simulink model "Experiment_Qcar_Nonlinear_MPC"  (R2024b)
settings: Solver=ode2  StartTime=0.0  StopTime=Tf  FixedStep=Ts2  RelTol=1e-3  EnableMultiTasking=on
values from neighbouring files (symbols this model uses):
  alpha_kalman = 0.9    [setup_FL_MPC.m]    (also in setup_NL_MPC.m; setup_backstepping.m)
  beta_kalman = 2    [setup_FL_MPC.m]    (also in setup_NL_MPC.m; setup_backstepping.m)
  kappa_kalman = 0    [setup_FL_MPC.m]    (also in setup_NL_MPC.m; setup_backstepping.m)
  l = 0.256    [setup_FL_MPC.m]    (also in setup_NL_MPC.m; setup_backstepping.m)
  N = 10    [setup_FL_MPC.m]    (also in setup_NL_MPC.m; setup_backstepping.m = 5)
  P0_kalman = diag([1e-5 1e-5 1e-6 1e-6])    [setup_FL_MPC.m]    (also in setup_NL_MPC.m; setup_backstepping.m)
  q0 = [x0;y0;theta0;0]    [setup_FL_MPC.m]    (also in setup_NL_MPC.m; setup_backstepping.m)
  Q_kalman = diag([0.001 0.001 0.1 1])    [setup_FL_MPC.m]    (also in setup_NL_MPC.m = diag([0.001 0.001 0.1 10]); setup_backstepping.m = diag([0.001 0.001 0.1 10]))
  Qhat = qz*eye(2*N)    [setup_FL_MPC.m]    (also in setup_NL_MPC.m = blkdiag(Qhat,Q))
  R_kalman = diag([2e-5 2e-5 0.0001 0.001])    [setup_FL_MPC.m]    (also in setup_NL_MPC.m = diag([2e-5 2e-5 0.0001 0.00001]); setup_backstepping.m = diag([2e-5 2e-5 0.0001 0.00001]))
  Rhat = qu*eye(2*N)    [setup_FL_MPC.m]    (also in setup_NL_MPC.m = blkdiag(Rhat,R))
  theta0 = vicon_data(6)    [setup_FL_MPC.m]    (also in setup_NL_MPC.m; setup_backstepping.m)
  Ts = 0.008    [setup_FL_MPC.m]    (also in setup_NL_MPC.m = 0.01; setup_backstepping.m = 0.1)
  Ts2 = Ts    (= 0.008)    [setup_FL_MPC.m]    (also in setup_NL_MPC.m = 0.01; setup_backstepping.m = 0.1)
  v1max = 1    [setup_FL_MPC.m]    (also in setup_NL_MPC.m; setup_backstepping.m)
  v2max = 10    [setup_FL_MPC.m]    (also in setup_NL_MPC.m; setup_backstepping.m)
  x0 = vicon_data(1)    [setup_FL_MPC.m]    (also in setup_NL_MPC.m; setup_backstepping.m)
  y0 = vicon_data(2)    [setup_FL_MPC.m]    (also in setup_NL_MPC.m; setup_backstepping.m)
undefined symbols (not defined in the file or in its folder): DiscIntNeverNeededParam, HIL
libraries: quarc_library x16, simulink x2, dspsigops x1, slpidlib x1
settings Model: SimulationMode=external  ExtModeTrigDuration=10000  Creator=mbohra  LastModifiedBy=tirio
settings SolverCC: AlgebraicLoopSolver=TrustRegion  PositivePriorityOrder=on  AutoInsertRateTranBlk=on
settings DataIOCC: SaveOutput=off  SignalLogging=off  DSMLogging=off  SaveTime=off  ReturnWorkspaceOutputs=off
settings OptimizationCC: ReuseModelBlockBuffer=off
settings DebuggingCC: UnconnectedInputMsg=warning  UnconnectedOutputMsg=warning  UnconnectedLineMsg=warning  ArithmeticOperatorsInVariantConditions=warning
settings HardwareCC: ProdBitPerLong=64  ProdLargestAtomicInteger=LongLong  ProdLargestAtomicFloat=Double  ProdLongLongMode=on  ProdHWDeviceType=ARM Compatible->ARM 64-bit (LP64)
settings ModelReferenceCC: EnableRefExpFcnMdlSchedulingChecks=on
settings SFSimCC: CustomCodeUndefinedFunction=UseInterfaceOnly
settings RTWCC: Description=QUARC Linux Nvidia Target (QCar) Using Toolchain  SystemTargetFile=quarc_linux_nvidia.tlc  TemplateMakefile=quarc_default_tmf  Toolchain=QUARC linux_nvidia | gmake (64-bit Windows)  BuildConfiguration=Faster Runs  GPUComputeCapability=3.5  DLArmComputeVersion=19.05
settings STFCustomTargetCC: TargetLangStandard=C99 (ISO)  ConcurrentExecutionCompliant=on  GRTInterface=on  UseToolchainInfoCompliant=on  SystemTargetFile=quarc_linux_nvidia.tlc
settings GRTTargetCC: ParMdlRefBuildCompliant=off  CompOptLevelCompliant=off  CombineOutputUpdateFcns=off  MatFileLogging=off  CPPClassGenCompliant=off  GRTInterface=on  ExtMode=on  ExtModeMexFile=quarc_comm  ExtModeMexArgs='-w -d /tmp -uri %u','tcpip://192.168.0.143:17001'

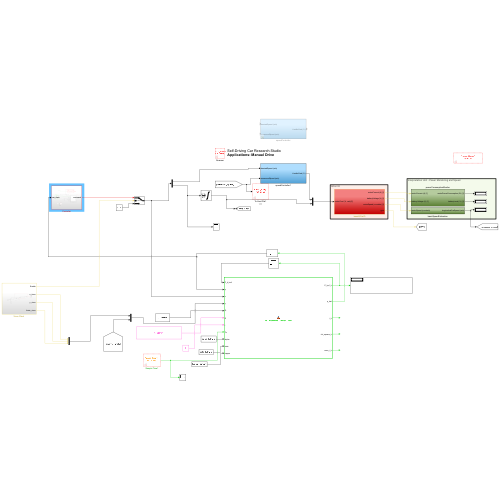
[thumbnail: Simulink's stored preview of the top-level diagram]
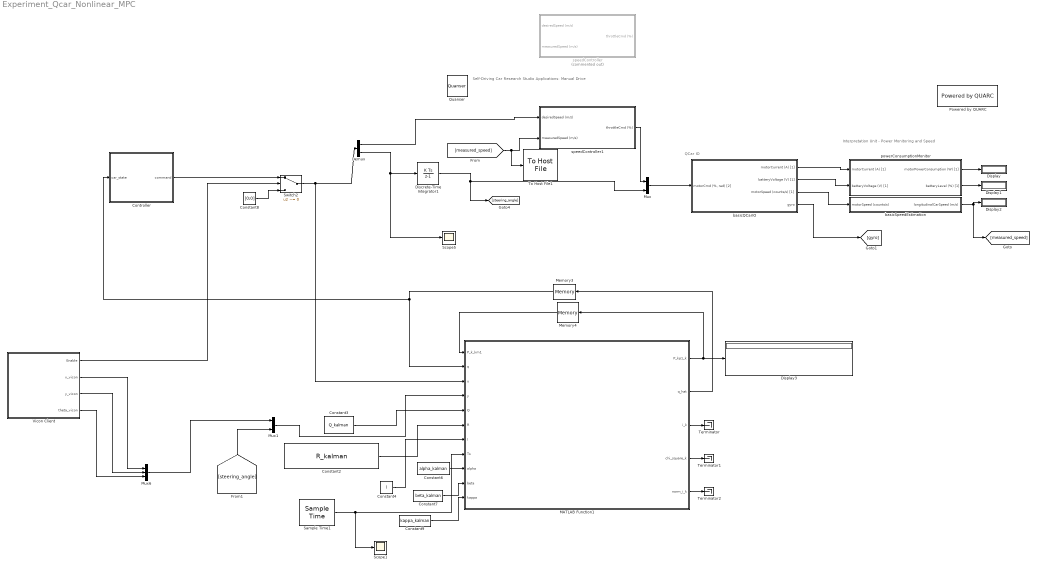
== system Experiment_Qcar_Nonlinear_MPC ==
  note: Interpretation Unit - Power Monitoring and Speed
  note: QCar IO
  note: Self-Driving Car Research Studio
      | Applications: Manual Drive
  Constant2 : Constant  Value=R_kalman
  Constant3 : Constant  Value=Q_kalman
  Constant4 : Constant  Value=l
  Constant6 : Constant  Value=alpha_kalman
  Constant7 : Constant  Value=beta_kalman
  Constant8 : Constant  Value=[0;0]
  Constant9 : Constant  Value=kappa_kalman
  Controller : Subsystem
  Demux : Demux  Outputs=2
  Discrete-Time Integrator1 : DiscreteIntegrator  SampleTime=Ts  LimitOutput=on  UpperSaturationLimit=0.6  LowerSaturationLimit=-0.6  ICPrevOutput=DiscIntNeverNeededParam  ICPrevScaledInput=DiscIntNeverNeededParam
  Display{,1..3} (4 alike) : Display
  MATLAB Function1 : MATLAB Function  TreatAsAtomicUnit=on
  Memory3 : Memory  InitialCondition=q0  InheritSampleTime=on
  Memory4 : Memory  InitialCondition=P0_kalman  InheritSampleTime=on
  Mux : Mux  Inputs=2
  Mux1 : Mux  Inputs=2
  Mux6 : Mux  Inputs=3
  Powered by QUARC : quarc_library/Logos/Powered by QUARC
  Quanser : quarc_library/Logos/Quanser
  Sample Time1 : quarc_library/Sources/Time/Sample Time  Priority=-99  sample_time=Ts
  Scope1 : Scope
  Scope5 : Scope
  Switch2 : Switch  Criteria=u2 ~= 0  SaturateOnIntegerOverflow=off  InputSameDT=off
  Terminator : Terminator
  Terminator1 : Terminator
  Terminator2 : Terminator
  To Host File1 : quarc_library/Sinks/To Host/To Host File  file_name=car_speed_NL_MPC2.mat  variable_name=v_car3  decimation=1  sample_time=-1  file_format=MAT-file v.4  options=No header or footer  append=off  final_file_name=car_speed_NL_MPC2.mat  bitrate=2000000
  "Vicon Client " : Subsystem
  basicQCarIO : Subsystem
  basicSpeedEstimation : Subsystem
  powerConsumptionMonitor : Subsystem
  speedController : Subsystem  Commented=on
  speedController1 : Subsystem
  wires:
  basicQCarIO/3(motorSpeed (counts/s) [1]) -> basicSpeedEstimation/1(motorSpeed (counts/s))
  basicQCarIO/1(motorCurrent (A) [1]) -> powerConsumptionMonitor/1(motorCurrent (A) [1])
  basicQCarIO/2(batteryVoltage (V) [1]) -> powerConsumptionMonitor/2(batteryVoltage (V) [1])
  powerConsumptionMonitor/2(batteryLevel (%) [1]) -> Display1/1
  powerConsumptionMonitor/1(motorPowerConsumption (W) [1]) -> Display/1
  Mux/1 -> basicQCarIO/1("motorCmd (%, rad) [2]")
  basicSpeedEstimation/1(longitudinalCarSpeed (m/s)) -> Display2/1, [measured_speed]
  [measured_speed] -> To Host File1/1, speedController1/2(measuredSpeed (m/s))
  speedController1/1(throttleCmd (%)) -> Mux/1
  Demux/2 -> Scope5/1, Discrete-Time Integrator1/1
  Sample Time1/1 -> Scope1/1, MATLAB Function1/8(Ts)
  Switch2/1 -> MATLAB Function1/3(u), Demux/1
  Controller/1(command) -> Switch2/1
  Constant8/1 -> Switch2/3
  MATLAB Function1/2(q_hat) -> Memory3/1
  MATLAB Function1/1(P_kp1_k) -> Display3/1, Memory4/1
  Memory4/1 -> MATLAB Function1/1(P_k_km1)
  Constant3/1 -> MATLAB Function1/5(Q)
  Constant2/1 -> MATLAB Function1/6(R)
  Constant4/1 -> MATLAB Function1/7(l)
  "Vicon Client "/1(Enable) -> Switch2/2
  "Vicon Client "/2(x_vicon) -> Mux6/1
  "Vicon Client "/3(y_vicon) -> Mux6/2
  "Vicon Client "/4(theta_vicon) -> Mux6/3
  Mux1/1 -> MATLAB Function1/4(y)
  Constant6/1 -> MATLAB Function1/9(alpha)
  Constant7/1 -> MATLAB Function1/10(beta)
  Constant9/1 -> MATLAB Function1/11(kappa)
  Mux6/1 -> Mux1/1
  [steering_angle] -> Mux1/2
  Memory3/1 -> MATLAB Function1/2(q), Controller/1(car_state)
  basicQCarIO/4(gyro) -> [gyro]
  Demux/1 -> speedController1/1(desiredSpeed (m/s))
  Discrete-Time Integrator1/1 -> Mux/2, [steering_angle]
  MATLAB Function1/3(i_k) -> Terminator/1
  MATLAB Function1/4(chi_square_k) -> Terminator1/1
  MATLAB Function1/5(norm_i_k) -> Terminator2/1

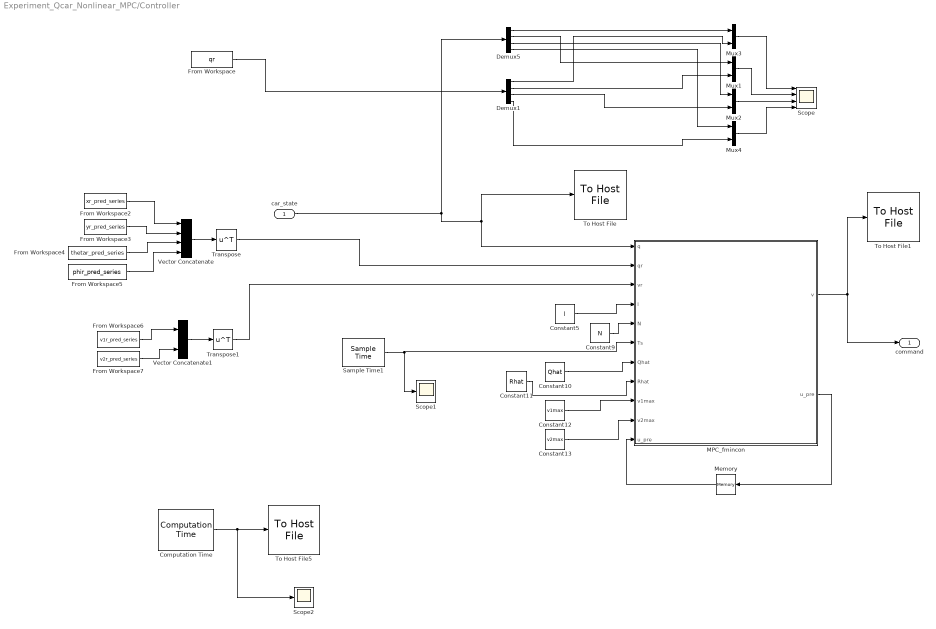
== system Experiment_Qcar_Nonlinear_MPC/Controller ==
  car_state : Inport
  Computation Time : quarc_library/Sources/Time/Computation Time  sample_time=qc_get_step_size  use_model=on  use_cpu_time=on
  Constant10 : Constant  Value=Qhat
  Constant11 : Constant  Value=Rhat
  Constant12 : Constant  Value=v1max
  Constant13 : Constant  Value=v2max
  Constant5 : Constant  Value=l
  Constant9 : Constant  Value=N
  Demux1 : Demux
  Demux5 : Demux
  From Workspace : FromWorkspace  VariableName=qr  SampleTime=Ts
  From Workspace2 : FromWorkspace  VariableName=xr_pred_series  SampleTime=Ts
  From Workspace3 : FromWorkspace  VariableName=yr_pred_series  SampleTime=Ts
  From Workspace4 : FromWorkspace  VariableName=thetar_pred_series  SampleTime=Ts
  From Workspace5 : FromWorkspace  VariableName=phir_pred_series  SampleTime=Ts
  From Workspace6 : FromWorkspace  VariableName=v1r_pred_series  SampleTime=Ts
  From Workspace7 : FromWorkspace  VariableName=v2r_pred_series  SampleTime=Ts
  MPC_fmincon : MATLAB Function  TreatAsAtomicUnit=on
  Memory : Memory  InitialCondition=zeros(2*N,1)
  Mux{1..4} (4 alike) : Mux  Inputs=2
  Sample Time1 : quarc_library/Sources/Time/Sample Time  Priority=-99  sample_time=Ts
  Scope : Scope  NumInputPorts=4
  Scope1 : Scope
  Scope2 : Scope
  To Host File : quarc_library/Sinks/To Host/To Host File  file_name=q_car_NL_MPC2.mat  variable_name=q_car3  decimation=1  sample_time=-1  file_format=MAT-file v.4  options=No header or footer  append=off  final_file_name=q_car_NL_MPC2.mat  bitrate=2000000
  To Host File1 : quarc_library/Sinks/To Host/To Host File  file_name=control_inputs_NL_MPC2.mat  variable_name=u_fb3  decimation=1  sample_time=-1  file_format=MAT-file v.4  options=No header or footer  append=off  final_file_name=control_inputs_NL_MPC2.mat  bitrate=2000000
  To Host File5 : quarc_library/Sinks/To Host/To Host File  file_name=CPU_time_NL_MPC_N10.mat  variable_name=cpu_time_NL_N10  decimation=1  sample_time=-1  file_format=MAT-file v.4  options=No header or footer  append=off  final_file_name=CPU_time_NL_MPC_N10.mat  bitrate=2000000
  Transpose : Math  Operator=transpose
  Transpose1 : Math  Operator=transpose
  Vector Concatenate : Concatenate  NumInputs=4  Mode=Multidimensional array  ConcatenateDimension=2
  Vector Concatenate1 : Concatenate  Mode=Multidimensional array  ConcatenateDimension=2
  command : Outport
  wires:
  MPC_fmincon/1(v) -> command/1, To Host File1/1
  From Workspace/1 -> Demux1/1
  car_state/1 -> To Host File/1, MPC_fmincon/1(q), Demux5/1
  Vector Concatenate/1 -> Transpose/1
  Vector Concatenate1/1 -> Transpose1/1
  Constant5/1 -> MPC_fmincon/4(l)
  Sample Time1/1 -> MPC_fmincon/6(Ts), Scope1/1
  From Workspace2/1 -> Vector Concatenate/1
  From Workspace3/1 -> Vector Concatenate/2
  From Workspace4/1 -> Vector Concatenate/3
  From Workspace5/1 -> Vector Concatenate/4
  From Workspace6/1 -> Vector Concatenate1/1
  From Workspace7/1 -> Vector Concatenate1/2
  Transpose/1 -> MPC_fmincon/2(qr)
  Transpose1/1 -> MPC_fmincon/3(vr)
  Demux5/3 -> Mux2/1
  Demux1/3 -> Mux2/2
  Mux1/1 -> Scope/2
  Demux1/4 -> Mux4/2
  Demux5/1 -> Mux3/1
  Demux5/2 -> Mux1/1
  Mux4/1 -> Scope/4
  Demux1/2 -> Mux1/2
  Demux5/4 -> Mux4/1
  Mux2/1 -> Scope/3
  Demux1/1 -> Mux3/2
  Mux3/1 -> Scope/1
  Constant13/1 -> MPC_fmincon/10(v2max)
  Constant9/1 -> MPC_fmincon/5(N)
  Constant12/1 -> MPC_fmincon/9(v1max)
  Constant10/1 -> MPC_fmincon/7(Qhat)
  Constant11/1 -> MPC_fmincon/8(Rhat)
  MPC_fmincon/2(u_pre) -> Memory/1
  Memory/1 -> MPC_fmincon/11("u_pre ")
  Computation Time/1 -> Scope2/1, To Host File5/1

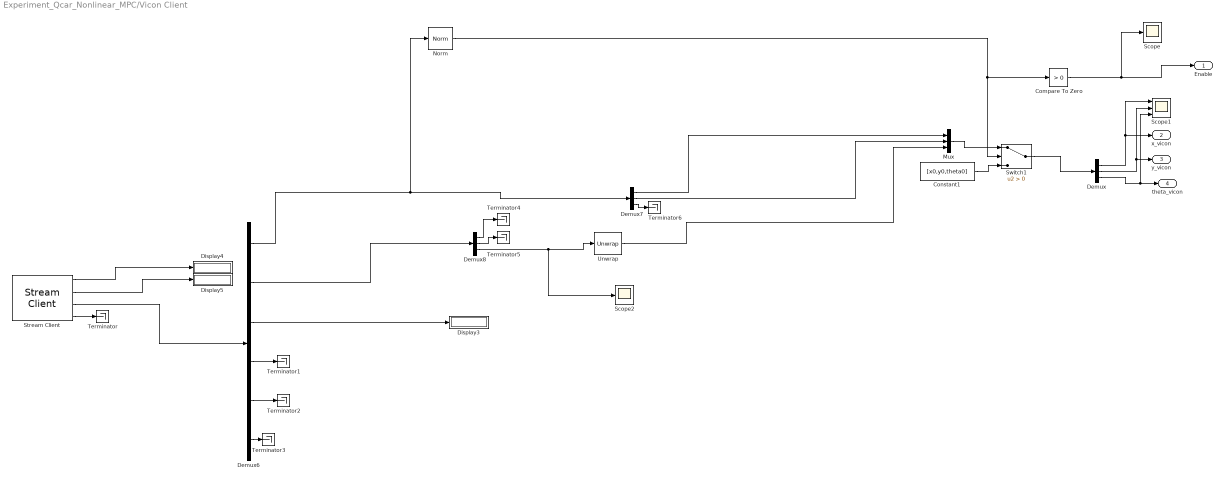
== system Experiment_Qcar_Nonlinear_MPC/Vicon Client  ==
  Compare To Zero : simulink/Logic and Bit Operations/Compare To Zero  relop=>  OutDataTypeStr=boolean
  Constant1 : Constant  Value=[x0,y0,theta0]
  Demux : Demux  Outputs=3
  Demux6 : Demux  Outputs=[3 3 1 3 3 1]
  Demux7 : Demux  Outputs=3
  Demux8 : Demux  Outputs=3
  Display3 : Display
  Display4 : Display
  Display5 : Display
  Mux : Mux  Inputs=3
  Norm : quarc_library/Math Operations/Vectors/Norm
      settings: SourceProductName=QUARC Targets
  Scope : Scope
  Scope1 : Scope  NumInputPorts=3
  Scope2 : Scope
  Stream Client : quarc_library/Communications/Basic/Stream Client  uri_source=Specify via dialog (do not evaluate)  uri=tcpip://192.168.0.5:18099  send_buffer_size=1460  receive_buffer_size=1460  byte_order=little endian (Intel - LSB first)  optimization=Minimum latency  send_options=Do not send data  receive_options=Receive most recent data  default_value=zeros(1,14)  sample_time=Ts  active=off  implementation=Use blocking I/O in a separate thread  send_fifo_size=1000  receive_fifo_size=1000  send_priority=0  receive_priority=0  send_dimensions=off  receive_dimensions=off  max_dimensions=-1  data_type=Inherited via back propagation  type_expr=BusObject
      settings: AttributesFormatString="\"tcpip://192.168.0.5:18099\""
  Switch1 : Switch  Criteria=u2 > Threshold  SaturateOnIntegerOverflow=off  InputSameDT=off
  Terminator{,1..6} (7 alike) : Terminator
  Unwrap : dspsigops/Unwrap  tol=pi  InputProcessing=Columns as channels (frame based)  running=off
  Enable : Outport
  x_vicon : Outport  Port=2
  y_vicon : Outport  Port=3
  theta_vicon : Outport  Port=4
  wires:
  Compare To Zero/1 -> Scope/1, Enable/1
  Mux/1 -> Switch1/1
  Switch1/1 -> Demux/1
  Demux8/2 -> Terminator5/1
  Stream Client/4 -> Terminator/1
  Demux6/3 -> Display3/1
  Demux6/4 -> Terminator1/1
  Stream Client/1 -> Display4/1
  Norm/1 -> Compare To Zero/1, Switch1/2
  Demux6/6 -> Terminator3/1
  Demux7/3 -> Terminator6/1
  Demux8/1 -> Terminator4/1
  Stream Client/3 -> Demux6/1
  Demux8/3 -> Scope2/1, Unwrap/1
  Demux7/1 -> Mux/1
  Stream Client/2 -> Display5/1
  Unwrap/1 -> Mux/3
  Demux/1 -> Scope1/1, x_vicon/1
  Demux6/1 -> Norm/1, Demux7/1
  Demux6/2 -> Demux8/1
  Demux6/5 -> Terminator2/1
  Demux7/2 -> Mux/2
  Demux/3 -> Scope1/3, theta_vicon/1
  Demux/2 -> Scope1/2, y_vicon/1
  Constant1/1 -> Switch1/3

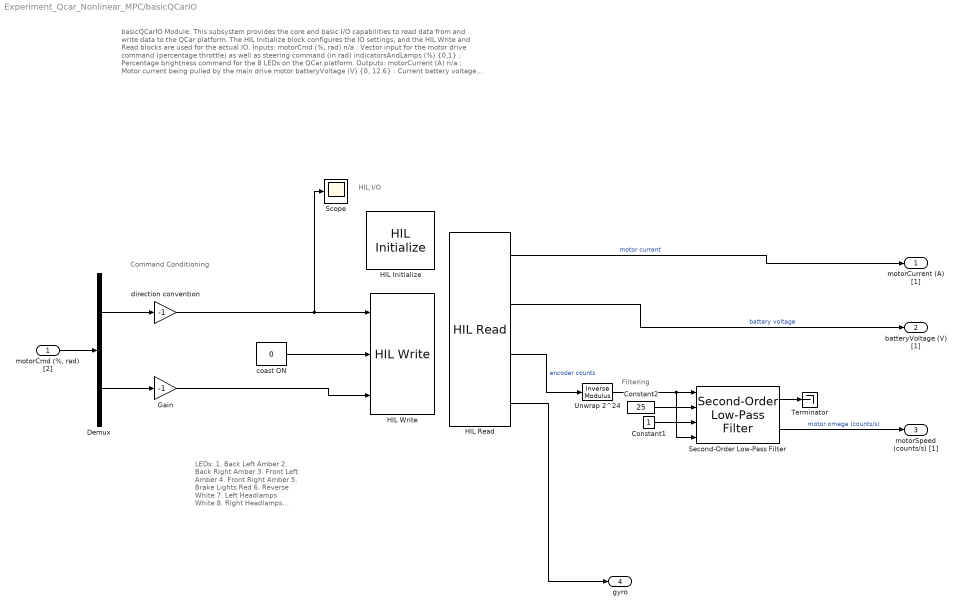
== system Experiment_Qcar_Nonlinear_MPC/basicQCarIO ==
  note: Filtering
  note: basicQCarIO Module:
      |
      | This subsystem provides the core and basic I/O capabilities to read data from and write data to the QCar platform. The HIL Initialize block configures the IO settings, and the HIL Write and Read blocks are used for the actual IO.
      |
      | Inputs:
      | motorCmd (%, rad) n/a : Vector input for the motor drive command (percentage throttle) as well as steering command (in rad)
      | indicatorsAndLamps (%) {0,1} : Percentage brightness command for the 8 LEDs on the QCar platform.
      |
      | Outputs:
      | motorCurrent (A) n/a : Motor current being pulled by the main drive motor
      | batteryVoltage (V) {0, 12.6} : Current battery voltage reading
      | motorSpeed (counts/s) n/a : Drive motor speed measured using an encoder (do not confuse with wheel speed as this measurement is at the drive shaft)
  note: Command Conditioning
  note: HIL I/O
  note: LEDs:
      | 1. Back Left Amber
      | 2. Back Right Amber
      | 3. Front Left Amber
      | 4. Front Right Amber
      | 5. Brake Lights Red
      | 6. Reverse White
      | 7. Left Headlamps White
      | 8. Right Headlamps White
  "motorCmd (%, rad) [2]" : Inport
  Constant1 : Constant
  Constant2 : Constant  Value=25
  Demux : Demux  Outputs=2
  Gain : Gain  Gain=-1
  HIL Initialize : quarc_library/Data Acquisition/Generic/Configuration/HIL Initialize  object_name=HIL-1  board_type=qcar  board_number=0  board_options=gyro_fs=250;gyro_rate=64;accel_fs=2;accel_rate=62.5;mag_rate=20;mag_xy=47;mag_z=83;enc1_dir=0;enc2_dir=0;enc3_dir=0;enc4_dir=0;pwm1_dshot=0;pwm2_dshot=0;pwm3_dshot=0;pwm4_dshot=0;pwm5_dshot=0;pwm6_dshot=0;pwm7_dshot=0;steer_bias=0.05;motor_limit=0.3;  exclusive=off  active=on  hardware_clocks=[]  clock_modes=[]  initial_clock_frequencies=[]  set_clock_params_at_start=off  set_clock_params_at_switch_in=off  set_clock_frequencies_at_start=off  set_clock_frequencies_at_switch_in=off  analog_input_channels=[0:6]  analog_input_configurations=[]  analog_input_maximums=[3.3]  analog_input_minimums=[0]  set_analog_input_params_at_start=off  set_analog_input_params_at_switch_in=off  analog_output_channels=[]  analog_output_maximums=[]  analog_output_minimums=[]  initial_analog_outputs=[]  final_analog_outputs=[]  watchdog_analog_outputs=[]  set_analog_output_params_at_start=off  set_analog_output_params_at_switch_in=off  set_analog_outputs_at_start=off  set_analog_outputs_at_switch_in=off  set_analog_outputs_at_terminate=off  set_analog_outputs_at_switch_out=off  set_analog_outputs_on_watchdog=off  digital_input_channels=[24:43]  digital_output_channels=[40]  digital_output_configuration=[]  initial_digital_outputs=[0]  final_digital_outputs=[1]  watchdog_digital_outputs=[]  set_digital_output_params_at_start=off  set_digital_output_params_at_switch_in=off  set_digital_outputs_at_start=on  set_digital_outputs_at_switch_in=off  set_digital_outputs_at_terminate=on  set_digital_outputs_at_switch_out=off  set_digital_outputs_on_watchdog=off  encoder_channels=[0:4]  quadrature=[4 4]  encoder_filter_frequency=100e6/1  initial_encoder_counts=[0]  set_encoder_params_at_start=on  set_encoder_params_at_switch_in=off  set_encoder_counts_at_start=on  set_encoder_counts_at_switch_in=off  pwm_channels=[0:7]  pwm_modes=[0 0]  pwm_frequency=150e6/4096  pwm_configuration=[0]  pwm_alignment=[0]  pwm_polarity=[1]  pwm_leading_deadband=[]  pwm_trailing_deadband=[]  initial_pwm_outputs=[0]  final_pwm_outputs=[0]  watchdog_pwm_outputs=[0]  set_pwm_params_at_start=on  set_pwm_params_at_switch_in=off  set_pwm_outputs_at_start=on  set_pwm_outputs_at_switch_in=off  set_pwm_outputs_at_terminate=on  set_pwm_outputs_at_switch_out=off  set_pwm_outputs_on_watchdog=off  other_output_channels=[1000, 11000:11011]  initial_other_outputs=[0]  final_other_outputs=[0]  watchdog_other_outputs=[]  set_other_outputs_at_start=on  set_other_outputs_at_switch_in=off  set_other_outputs_at_terminate=on  set_other_outputs_at_switch_out=off  set_other_outputs_on_watchdog=off
  HIL Read : quarc_library/Data Acquisition/Generic/Immediate I//O/HIL Read  object_name=HIL-1  analog_channels=[5:6]  encoder_channels=[0]  digital_channels=[]  other_channels=[3002]  sample_time=qc_get_step_size  active=on  vector_output=off  data_type_mode=Inherit via back propagation  encoder_data_type=double  digital_data_type=boolean
  HIL Write : quarc_library/Data Acquisition/Generic/Immediate I//O/HIL Write  object_name=HIL-1  analog_channels=[]  pwm_channels=[0]  digital_channels=[40]  other_channels=[1000 ]  sample_time=-1  active=off  vector_input=on
  Scope : Scope
  Second-Order Low-Pass Filter : quarc_library/Continuous/Second-Order Low-Pass Filter  params_source=External (input ports)  input_width=1  input_zeta=1  input_init=0
  Terminator : Terminator
  Unwrap 2^24 : quarc_library/Discontinuities/Inverse Modulus  modulus=16777215  output_derivative=off  output_revolutions=off  max_x=Inf  min_x=-Inf
  coast ON : Constant  Value=0
  direction convention : Gain  Gain=-1
  motorCurrent (A) [1] : Outport  VectorParamsAs1DForOutWhenUnconnected=off
  batteryVoltage (V) [1] : Outport  Port=2  VectorParamsAs1DForOutWhenUnconnected=off
  motorSpeed (counts/s) [1] : Outport  Port=3  VectorParamsAs1DForOutWhenUnconnected=off
  gyro : Outport  Port=4
  wires:
  Constant2/1 -> Second-Order Low-Pass Filter/2
  Unwrap 2^24/1 -> Second-Order Low-Pass Filter/1, Second-Order Low-Pass Filter/4
  Demux/2 -> Gain/1
  "motorCmd (%, rad) [2]"/1 -> Demux/1
  direction convention/1 -> Scope/1, HIL Write/1
  coast ON/1 -> HIL Write/2
  Second-Order Low-Pass Filter/1 -> Terminator/1
  Gain/1 -> HIL Write/3
  Second-Order Low-Pass Filter/2 -> motorSpeed (counts/s) [1]/1  "motor omega (counts/s)"
  Constant1/1 -> Second-Order Low-Pass Filter/3
  Demux/1 -> direction convention/1
  HIL Read/3 -> Unwrap 2^24/1  "encoder counts"
  HIL Read/1 -> motorCurrent (A) [1]/1  "motor current"
  HIL Read/2 -> batteryVoltage (V) [1]/1  "battery voltage"
  HIL Read/4 -> gyro/1

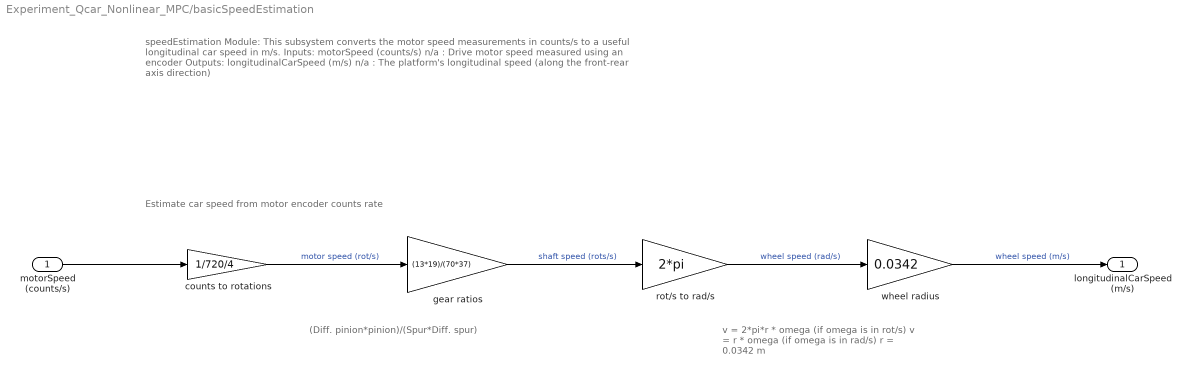
== system Experiment_Qcar_Nonlinear_MPC/basicSpeedEstimation ==
  note: speedEstimation Module:
      |
      | This subsystem converts the motor speed measurements in counts/s to a useful longitudinal car speed in m/s.
      |
      | Inputs:
      | motorSpeed (counts/s) n/a : Drive motor speed measured using an encoder
      |
      | Outputs:
      | longitudinalCarSpeed (m/s) n/a : The platform's longitudinal speed (along the front-rear axis direction)
  note: (Diff. pinion*pinion)/(Spur*Diff. spur)
  note: v = 2*pi*r * omega (if omega is in rot/s)
      | v = r * omega (if omega is in rad/s)
      | r = 0.0342 m
  note: Estimate car speed from motor encoder counts rate
  motorSpeed (counts/s) : Inport
  counts to rotations : Gain  Gain=1/720/4
  gear ratios : Gain  Gain=(13*19)/(70*37)
  rot/s to rad/s : Gain  Gain=2*pi
  wheel radius : Gain  Gain=0.0342
  longitudinalCarSpeed (m/s) : Outport  VectorParamsAs1DForOutWhenUnconnected=off
  wires:
  gear ratios/1 -> rot/s to rad/s/1  "shaft speed (rots/s)"
  wheel radius/1 -> longitudinalCarSpeed (m/s)/1  "wheel speed (m/s)"
  counts to rotations/1 -> gear ratios/1  "motor speed (rot/s)"
  rot/s to rad/s/1 -> wheel radius/1  "wheel speed (rad/s)"
  motorSpeed (counts/s)/1 -> counts to rotations/1

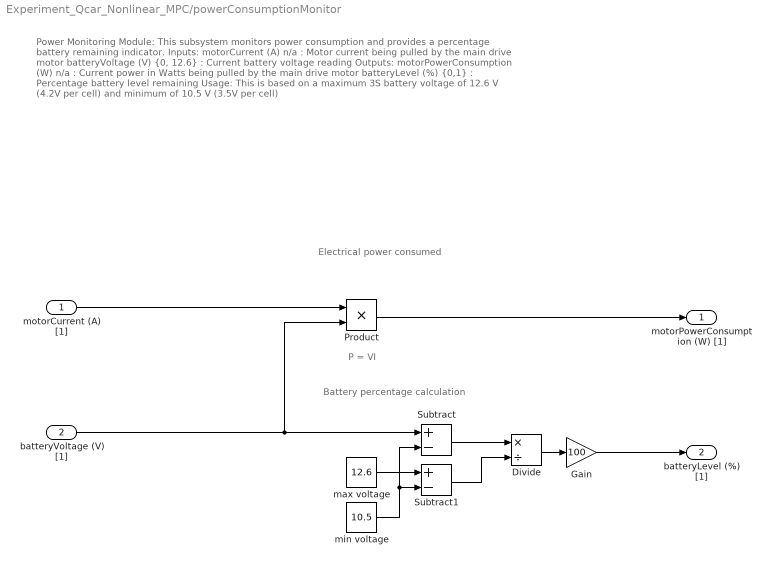
== system Experiment_Qcar_Nonlinear_MPC/powerConsumptionMonitor ==
  note: Battery percentage calculation
  note: P = VI
  note: Electrical
      | power
      | consumed
  note: Power Monitoring Module:
      |
      | This subsystem monitors power consumption and provides a percentage battery remaining indicator.
      |
      | Inputs:
      | motorCurrent (A) n/a : Motor current being pulled by the main drive motor
      | batteryVoltage (V) {0, 12.6} : Current battery voltage reading
      |
      | Outputs:
      | motorPowerConsumption (W) n/a : Current power in Watts being pulled by the main drive motor
      | batteryLevel (%) {0,1} : Percentage battery level remaining
      |
      | Usage:
      | This is based on a maximum 3S battery voltage of 12.6 V (4.2V per cell) and minimum of 10.5 V (3.5V per cell)
  motorCurrent (A) [1] : Inport
  batteryVoltage (V) [1] : Inport  Port=2
  Divide : Product  Inputs=*/
  Gain : Gain  Gain=100
  Product : Product
  Subtract : Sum  Inputs=+-
  Subtract1 : Sum  Inputs=+-
  max voltage : Constant  Value=12.6
  min voltage : Constant  Value=10.5
  motorPowerConsumption (W) [1] : Outport  VectorParamsAs1DForOutWhenUnconnected=off
  batteryLevel (%) [1] : Outport  Port=2  VectorParamsAs1DForOutWhenUnconnected=off
  wires:
  Divide/1 -> Gain/1
  Subtract1/1 -> Divide/2
  Gain/1 -> batteryLevel (%) [1]/1
  Product/1 -> motorPowerConsumption (W) [1]/1
  min voltage/1 -> Subtract/2, Subtract1/2
  motorCurrent (A) [1]/1 -> Product/1
  max voltage/1 -> Subtract1/1
  Subtract/1 -> Divide/1
  batteryVoltage (V) [1]/1 -> Subtract/1, Product/2

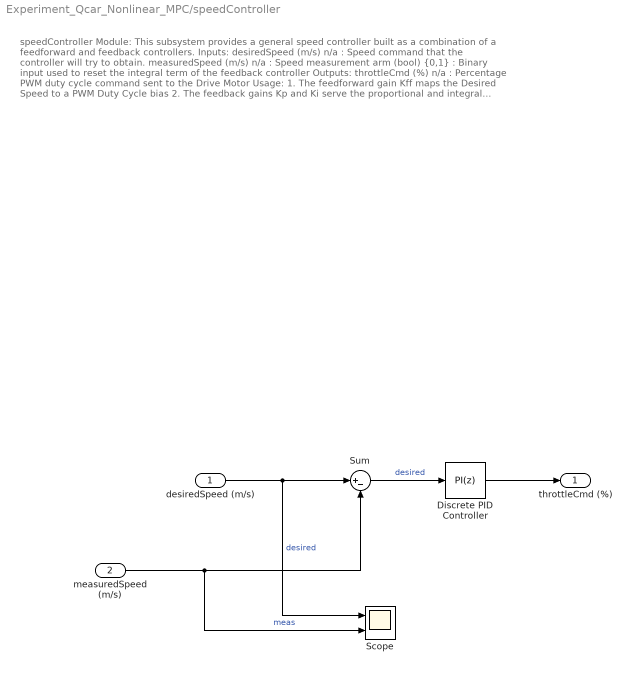
== system Experiment_Qcar_Nonlinear_MPC/speedController ==
  note: speedController Module:
      |
      | This subsystem provides a general speed controller built as a combination of a feedforward and feedback controllers.
      |
      | Inputs:
      | desiredSpeed (m/s) n/a : Speed command that the controller will try to obtain.
      | measuredSpeed (m/s) n/a : Speed measurement
      | arm (bool) {0,1} : Binary input used to reset the integral term of the feedback controller
      |
      | Outputs:
      | throttleCmd (%) n/a : Percentage PWM duty cycle command sent to the Drive Motor
      |
      | Usage:
      | 1. The feedforward gain Kff maps the Desired Speed to a PWM Duty Cycle bias
      | 2. The feedback gains Kp and Ki serve the proportional and integral terms to output corrections to the PWM Duty Cycle so as to regulate the desired speed.
  desiredSpeed (m/s) : Inport
  measuredSpeed (m/s) : Inport  Port=2
  Discrete PID Controller : slpidlib/PID Controller  Controller=PI  Form=Parallel  TimeDomain=Discrete-time  UseExternalTs=off  SampleTime=Ts2  IntegratorMethod=Forward Euler  FilterMethod=Forward Euler  ControllerParametersSource=internal  P=0.4  I=2*Ts2  UseKiTs=on  D=0  N=100  UseFilter=on  TunerSelectOption=Transfer Function Based (PID Tuner App)  InitialConditionSource=internal  InitialConditionForIntegrator=0  InitialConditionForFilter=0  DifferentiatorICPrevScaledInput=0  ExternalReset=none  TrackingMode=off  Kt=1  LimitOutput=on  SatLimitsSource=internal  UpperSaturationLimit=0.5  LowerSaturationLimit=-0.5  LinearizeAsGain=off  AntiWindupMode=back-calculation  Kb=1  LimitIntegrator=off  UpperIntegratorSaturationLimit=inf  LowerIntegratorSaturationLimit=-inf  POutMin=[]  POutMax=[]  IOutMin=[]  IOutMax=[]  DOutMin=[]  DOutMax=[]  NOutMin=[]  NOutMax=[]  SumOutMin=[]  SumOutMax=[]  SaturationOutMin=[]  SaturationOutMax=[]  PParamMin=[]  PParamMax=[]  IParamMin=[]  IParamMax=[]  DParamMin=[]  DParamMax=[]  NParamMin=[]  NParamMax=[]  KbParamMin=[]  KbParamMax=[]  KtParamMin=[]  KtParamMax=[]  KbOutMin=[]  KbOutMax=[]  KtOutMin=[]  KtOutMax=[]  IntegratorOutMin=[]  IntegratorOutMax=[]  FilterOutMin=[]  FilterOutMax=[]  SumI1OutMin=[]  SumI1OutMax=[]  SumI2OutMin=[]  SumI2OutMax=[]  SumI3OutMin=[]  SumI3OutMax=[]  SumI4OutMin=[]  SumI4OutMax=[]  SumDOutMin=[]  SumDOutMax=[]  DifferentiatorOutMin=[]  DifferentiatorOutMax=[]  FilterDiffOutCoefMin=[]  FilterDiffOutCoefMax=[]  ReciprocalOutMin=[]  ReciprocalOutMax=[]  SumDenOutMin=[]  SumDenOutMax=[]  SumNumOutMin=[]  SumNumOutMax=[]  DivideOutMin=[]  DivideOutMax=[]  UdiffTsProdOutMin=[]  UdiffTsProdOutMax=[]  NTsProdOutMin=[]  NTsProdOutMax=[]  UintegralTsProdOutMin=[]  UintegralTsProdOutMax=[]  UngainTsProdOutMin=[]  UngainTsProdOutMax=[]  ClampingZeroOutDataTypeStr=Inherit: Inherit via back propagation  ClampingZeroOutMin=[]  ClampingZeroOutMax=[]  FilterDenConstantOutDataTypeStr=Inherit: Inherit via back propagation  FilterDenConstantOutMin=[]  FilterDenConstantOutMax=[]  PCopyOutDataTypeStr=Inherit: Inherit via back propagation  PCopyOutMin=[]  PCopyOutMax=[]  NCopyOutDataTypeStr=Inherit: Inherit via back propagation  NCopyOutMin=[]  NCopyOutMax=[]  IntegratorContinuousStateAttributes=''  IntegratorStateMustResolveToSignalObject=off  IntegratorRTWStateStorageClass=Auto  FilterContinuousStateAttributes=''  FilterStateMustResolveToSignalObject=off  FilterRTWStateStorageClass=Auto  ParallelPVariant=InternalParameters  IdealPVariant=Disabled  IVariant=InternalParameters  DVariant=Disabled  IntegratorVariant=Discrete  SatVariant=Enabled  AWVariant=BackCalculation  PCopyVariant=Disabled  TRVariant=Disabled  FdbkBlocksVariant=Forward  IdealPFdbkVariant=Disabled  SatFdbkVariant=Disabled  DerivativeFilterVariant=Disabled  NVariant=Disabled  NCopyVariant=Disabled_SignalSpec  FilterICVariant=Disabled  IntegratorICVariant=InternalICs  ExternalResetVariant=Disabled  TRSumVariant=Passthrough  SumFdbkVariant=Disabled  SumVariant=Sum_PI  TsampFilterVariant=InternalTs  TsampNgainVariant=Passthrough  TsampIntegralVariant=Passthrough  ExternalSaturationOutDataTypeStr=Inherit: Same as second input
      settings: LibrarySourceBlock=simulink/Discrete/Discrete PID Controller
  Scope : Scope  NumInputPorts=2
  Sum : Sum  Inputs=|+-
  throttleCmd (%) : Outport  VectorParamsAs1DForOutWhenUnconnected=off
  wires:
  Discrete PID Controller/1 -> throttleCmd (%)/1
  measuredSpeed (m/s)/1 -> Sum/2, Scope/2  "meas"
  desiredSpeed (m/s)/1 -> Sum/1, Scope/1  "desired"
  Sum/1 -> Discrete PID Controller/1  "desired"

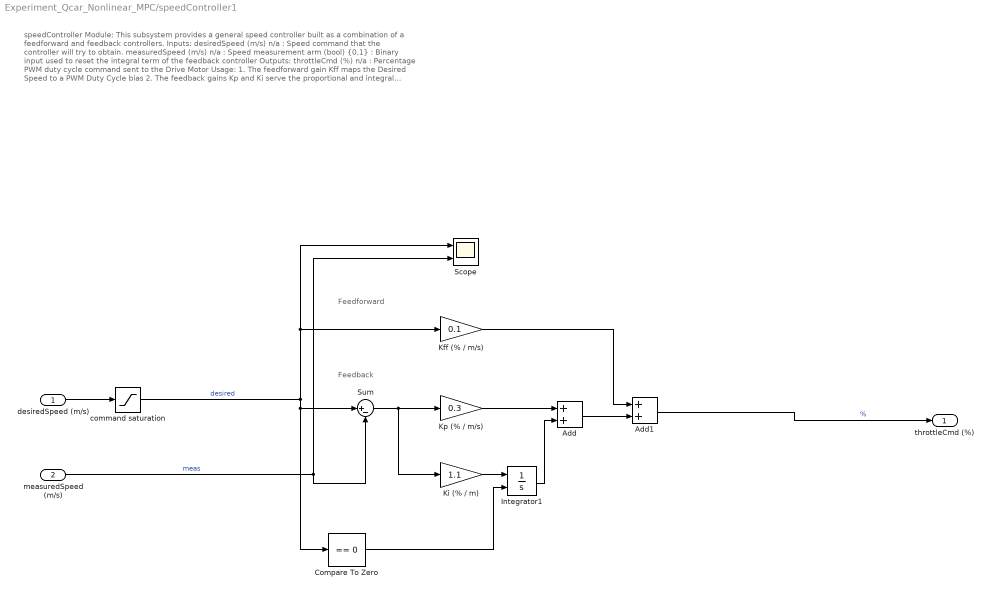
== system Experiment_Qcar_Nonlinear_MPC/speedController1 ==
  note: Feedforward
  note: Feedback
  note: speedController Module:
      |
      | This subsystem provides a general speed controller built as a combination of a feedforward and feedback controllers.
      |
      | Inputs:
      | desiredSpeed (m/s) n/a : Speed command that the controller will try to obtain.
      | measuredSpeed (m/s) n/a : Speed measurement
      | arm (bool) {0,1} : Binary input used to reset the integral term of the feedback controller
      |
      | Outputs:
      | throttleCmd (%) n/a : Percentage PWM duty cycle command sent to the Drive Motor
      |
      | Usage:
      | 1. The feedforward gain Kff maps the Desired Speed to a PWM Duty Cycle bias
      | 2. The feedback gains Kp and Ki serve the proportional and integral terms to output corrections to the PWM Duty Cycle so as to regulate the desired speed.
  desiredSpeed (m/s) : Inport
  measuredSpeed (m/s) : Inport  Port=2
  Add : Sum
  Add1 : Sum
  Compare To Zero : simulink/Logic and Bit Operations/Compare To Zero  relop===  OutDataTypeStr=boolean
  Integrator1 : Integrator  ExternalReset=either  LimitOutput=on  UpperSaturationLimit=0.4  LowerSaturationLimit=-0.4
  Kff (% / m/s) : Gain  Gain=0.1
  "Ki (% / m) " : Gain  Gain=1.1
  Kp (% / m/s) : Gain  Gain=0.3
  Scope : Scope  NumInputPorts=2
  Sum : Sum  Inputs=|+-
  command saturation : Saturate  UpperLimit=5  LowerLimit=-5
  throttleCmd (%) : Outport  VectorParamsAs1DForOutWhenUnconnected=off
  wires:
  command saturation/1 -> Compare To Zero/1, Sum/1, Kff (% / m/s)/1, Scope/1  "desired"
  measuredSpeed (m/s)/1 -> Sum/2, Scope/2  "meas"
  Add/1 -> Add1/2
  Add1/1 -> throttleCmd (%)/1  "%"
  Integrator1/1 -> Add/2
  Kp (% / m/s)/1 -> Add/1
  Compare To Zero/1 -> Integrator1/2
  Kff (% / m/s)/1 -> Add1/1
  Sum/1 -> "Ki (% / m) "/1, Kp (% / m/s)/1
  "Ki (% / m) "/1 -> Integrator1/1
  desiredSpeed (m/s)/1 -> command saturation/1

== matlab function Experiment_Qcar_Nonlinear_MPC/Controller/MPC_fmincon ==
  data: q input; v output; qr input; vr input; l input; N input; Ts input; Qhat input; Rhat input; v1max input; v2max input; u_pre input; u_pre output
function [v,u_pre]= MPC_fmincon_tracking_controller(q,qr,vr,l,N,Ts,Qhat,Rhat,v1max,v2max,u_pre)









%Set theoretic MPC online optimization


    function obj=obj_fun(u,q,qr,vr,l,Ts,Qhat,Rhat,N)


        %         qtilde=zeros(4*N,1);
        %
        %         qtilde(1:4,1)=q-qr(:,1);
        %
        %         qcurr=q;
        %
        %         for i=1:N-1
        %
        %
        %             qnext = qcurr +Ts*[cos(qcurr(3)) 0;
        %                 sin(qcurr(3)) 0;
        %                 tan(qcurr(4))/l 0;
        %                 0          1]*u(2*i-1:2*i);
        %
        %             qtilde(4*i+1:4*i+4,1)=qnext-qr(:,i+1);
        %
        %             qcurr=qnext;
        %
        %         end




        qtilde=zeros(4*N,1);

        qcurr=q;

        for i=1:N


            qnext = qcurr +Ts*[cos(qcurr(3)) 0;
                sin(qcurr(3)) 0;
                tan(qcurr(4))/l 0;
                0          1]*u(2*i-1:2*i);

            qtilde(4*i-3:4*i,1)=qnext-qr(:,i);

            qcurr=qnext;

        end





        Wr=zeros(2*N,1);

        for j=1:N
            Wr(2*(j-1)+1:2*j)=vr(:,j);
        end

        obj=qtilde'*Qhat*qtilde+(u)'*Rhat*(u);


    end







T=[-1 0; 0 -1; 1 0; 0 1];
% Hk=T/T_FL;
g=[v1max;v2max;v1max;v2max];



 H_constr=zeros(4*N,2*N);
 g_constr=zeros(4*N,1);

 for k=1:N

     H_constr(4*k-3:4*k,2*k-1:2*k)=T;
     g_constr(4*k-3:4*k,1)=g;

 end




options=optimoptions('fmincon','Display','off','Algorithm','sqp-legacy');

options.MaxIterations = 100;
options.ConstraintTolerance = 1.0e-6;
options.OptimalityTolerance = 1.0e-6;


usol = fmincon(@(u)obj_fun(u,q,qr,vr,l,Ts,Qhat,Rhat,N),u_pre,H_constr,g_constr,[],[],[],[],[],options);
u_pre=usol;
v=usol(1:2);



end

== matlab function Experiment_Qcar_Nonlinear_MPC/MATLAB Function1 ==
  data: P_k_km1 input; P_kp1_k output; q input; u input; q_hat output; y input; Q input; R input; l input; Ts input; alpha input; beta input; kappa input; i_k output; chi_square_k output; norm_i_k output
function [P_kp1_k,q_hat,i_k,chi_square_k,norm_i_k]= my_unscented_kalman_filter(P_k_km1,q,u,y,Q,R,l,Ts,alpha,beta,kappa)

%Calculate the Sigma points
M=4;
c=alpha^2*(M+kappa);

q_hat_i=zeros(M,2*M+1);

q_hat_i(:,1)=q;


Delta_x=real(sqrtm(c*P_k_km1));

for i=1:M
    q_hat_i(:,i+1)=q+Delta_x(:,i);
    q_hat_i(:,i+1+M)=q-Delta_x(:,i);
end


%Output of the sigma points
y_hat_i=q_hat_i(1:4,:);

%predicted measurement at time k
W_M=zeros(1,2*M+1);
W_M(1)=1-(M/(alpha^2*(M+kappa)));
W_M(2:2*M+1)=(1/(2*alpha^2*(M+kappa)));

y_k=zeros(4,1);

for i=1:2*M+1
    y_k=y_k+W_M(i)*y_hat_i(:,i);
end



%Estimate of the covariance of predicted measurement
W_c=zeros(1,2*M+1);
W_c(1)=(2-alpha^2+beta)-(M/(alpha^2*(M+kappa)));
W_c(2:2*M+1)=(1/(2*alpha^2*(M+kappa)));

P_y=zeros(4,4);

for i=1:2*M+1
    P_y=P_y+W_c(i)*(y_hat_i(:,i)-y_k)*(y_hat_i(:,i)-y_k)'+R;
end


%%Estimate of the cross-covariance between predicted x and y
P_xy=zeros(4,4);
for i=1:2*M+1
    P_xy=P_xy+(1/(2*alpha^2*(M+kappa)))*(q_hat_i(:,i)-q)*(y_hat_i(:,i)-y_k)';
end


%Kalman gain
K=P_xy/(P_y);

q_k_k = q+K*(y-y_k);
P_k_k = P_k_km1 -K*P_y*K';


% State prediction and state estimation error covariance

q_hat_i_k_k=zeros(4,2*M+1);
q_hat_i_k_k(:,1)=q_k_k;

Delta_x=real(sqrtm(c*P_k_k));

for i=1:M
    q_hat_i_k_k(:,i+1)=q_k_k+Delta_x(:,i);
    q_hat_i_k_k(:,i+1+M)=q_k_k-Delta_x(:,i);
end


%Predicted state for each sigma point

q_hat_kp1_k=zeros(4,2*M+1);

for i=1:2*M+1
    q_hat_kp1_k(:,i)=q_hat_i_k_k(:,i)+Ts*[cos(q_hat_i_k_k(3,i)) 0;
        sin(q_hat_i_k_k(3,i)) 0;
        tan(q_hat_i_k_k(4,i))/l 0;
        0          1]*u;


    %Steering angle saturation
    if q_hat_kp1_k(4,i)>0.6

        q_hat_kp1_k(4,i)=0.6;

    elseif q_hat_kp1_k(4,i)<-0.6
        q_hat_kp1_k(4,i)=-0.6;

    end

end


%Predicted state k+1 at time k
q_hat=zeros(4,1);
for i=1:2*M+1
    q_hat=q_hat + W_M(i)*q_hat_kp1_k(:,i);
end

%Covariance of the predicted state
P_kp1_k=zeros(4,4);

for i=1:2*M+1
    P_kp1_k=P_kp1_k+W_c(i)*(q_hat_kp1_k(:,i)-q_hat)*(q_hat_kp1_k(:,i)-q_hat)'+Q;
end


i_k=y-q_hat;
S_k=P_k_km1+R;

norm_i_k=inv(sqrtm(S_k))*i_k;

chi_square_k=i_k'*inv(S_k)*i_k;
